simulink model "sim4"  (Simulink 8.1)
settings: Solver=ode15s  StartTime=0.0  StopTime=10  RelTol=1e-3
libraries: cstblocks x2
settings Model: Creator=gscorlet  LastModifiedBy=Anton Korniienko
settings DataIOCC: Refine=10
settings OptimizationCC: BooleanDataType=off  InitFltsAndDblsToZero=on
settings DebuggingCC: SaveWithParameterizedLinksMsg=none  SignalResolutionControl=TryResolveAllWithWarning  SolverPrmCheckMsg=none  MultiTaskDSMMsg=warning  MultiTaskCondExecSysMsg=none  StrictBusMsg=None
settings HardwareCC: TargetUnknown=on
settings RTWCC: IncludeERTFirstTime=on

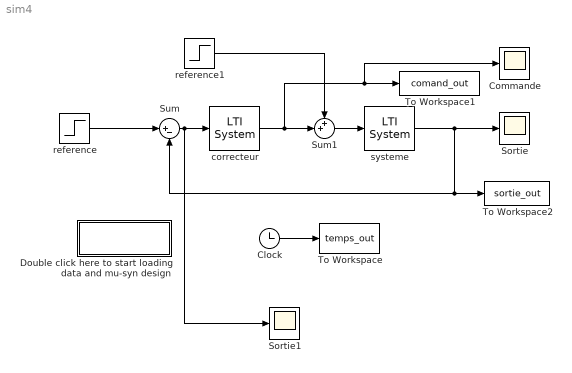
== system sim4 ==
  Clock : Clock
  Commande : Scope
  Double click here to start loading data and mu-syn design : Subsystem
      settings: OpenFcn=figure(FIG_SIM);subplot(211); plot(temps_out, sortie_out, 'r'); grid on; title('Sortie'); subplot(212); plot(temps_out, comand_out, 'r-'); title('Commande'); grid on;
      mask Display: disp('Plot figure')
  Sortie : Scope
  Sortie1 : Scope
      settings: SaveName=ScopeData2
  Sum : Sum  Inputs=|+-  SaturateOnIntegerOverflow=on  InputSameDT=on  OutDataTypeStr=Inherit: Same as first input
  Sum1 : Sum  Inputs=++|  SaturateOnIntegerOverflow=on  InputSameDT=on  OutDataTypeStr=Inherit: Same as first input
  To Workspace : ToWorkspace  VariableName=temps_out  SampleTime=-1
  To Workspace1 : ToWorkspace  VariableName=comand_out  SampleTime=-1
  To Workspace2 : ToWorkspace  VariableName=sortie_out  SampleTime=-1
  correcteur : cstblocks/LTI System  sys=ss_k  IC=0
  reference : Step  Time=0  SampleTime=0
  reference1 : Step  Time=0.5  SampleTime=0
  systeme : cstblocks/LTI System  sys=f_sys  IC=[]
  wires:
  Sum/1 -> correcteur/1, Sortie1/1
  Sum1/1 -> systeme/1
  correcteur/1 -> Sum1/2, To Workspace1/1, Commande/1
  Clock/1 -> To Workspace/1
  reference/1 -> Sum/1
  reference1/1 -> Sum1/1
  systeme/1 -> Sum/2, To Workspace2/1, Sortie/1

== system sim4/Double click here to start loading data and mu-syn design ==
